simulink model "Questao1_1"  (R2023b)
settings: Solver=VariableStepAuto  StartTime=0.0  StopTime=0.1  RelTol=1e-3
undefined symbols (not defined in the file): b, f_final, f_inicial, k, m, t_inicial

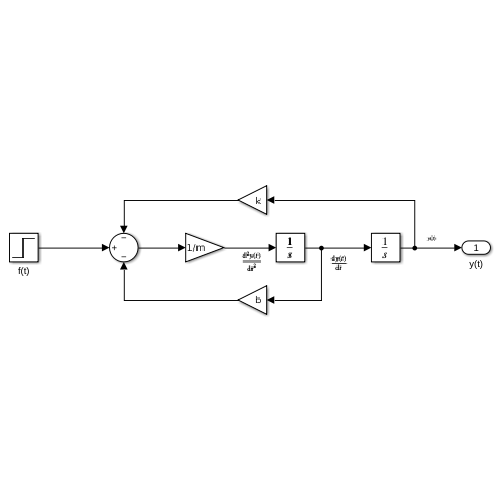
[thumbnail: Simulink's stored preview of the top-level diagram]
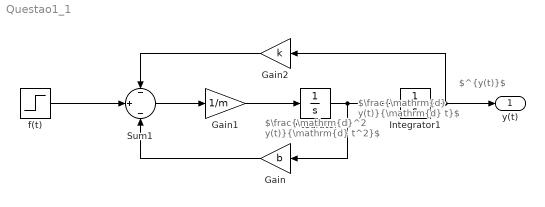
== system Questao1_1 ==
  note: $^{y(t)}$
  note: $\frac{\mathrm{d} y(t)}{\mathrm{d} t}$
  note: $\frac{\mathrm{d}^2 y(t)}{\mathrm{d} t^2}$
  Gain : Gain  Gain=b
  Gain1 : Gain  Gain=1/m
  Gain2 : Gain  Gain=k
  Integrator : Integrator
  Integrator1 : Integrator
  Sum1 : Sum  Inputs=-|+|-
  f(t) : Step  Time=t_inicial  Before=f_inicial  After=f_final  SampleTime=0
  y(t) : Outport
  wires:
  f(t)/1 -> Sum1/2
  Gain1/1 -> Integrator/1
  Integrator/1 -> Gain/1, Integrator1/1
  Integrator1/1 -> Gain2/1, y(t)/1
  Gain2/1 -> Sum1/1
  Gain/1 -> Sum1/3
  Sum1/1 -> Gain1/1
